simulink library "libbha_kinetic_cc"  (R2013b)
settings: Solver=FixedStepDiscrete  StartTime=0.0  StopTime=Inf  FixedStep=0.004  RelTol=1e-3
PostLoadFcn:
  | , if any(exist('dsrtsu_mdlpostloadfcn', 'file') == [2, 3, 6]), try dsrtsu_mdlpostloadfcn('Execute', bdroot); catch fprintf('Error in PostLoadFcn (dsrtsu_mdlpostloadfcn) for model "%s":\n %s\n', bdroot, lasterr); end, end,
libraries: libbha_parts_bellows x2
(part 2 of 4)

== matlab function libbha_kinetic_cc/lib_kinm_ext_S1 ==
  data: q input size=[3,1]; dq input size=[3,1]; H_1b_w input size=[4,4]; PAR_ell_ib input size=1; PAR_ell_ih input size=1; PAR_r_Bi input size=1; H_1h_w output size=[4,4]; dHdq_1h_w output size=[12,4]; dHPdq_1h_w output size=[12,4]; r_Bik_1h output size=[4,3]
% Kinetic Simulation
function [H_1h_w, dHdq_1h_w, dHPdq_1h_w, r_Bik_1h ] =  ksim_ext(q,dq, H_1b_w, PAR_ell_ib, PAR_ell_ih, PAR_r_Bi)

  
    
    % Änderungen zut alten Version:
    % - Rückrechnung mit Offsets der 4. Dimension der Homogenen Transformation (HOxx)
    % - richtige Saturierung des Ausgangsdrucks (optional)
    % - Tensordarstellung vermieden (Vektoren oder Matrizen sofern möglich), daher auch mehr getrennte Variablen
    % - Zusammenfassung bei Berechnungen unter Ausnutzung von 0-Einträgen (schwerer lesbar und weniger allgemein, dafür schneller zu rechnen)


%% Zustands- und Ableitungsberechnung der Homogenen Transformationen
    
    k                 = calc_k_i(q(1), q(2), q(3), PAR_r_Bi(1));
    
    dkdq_S1              = calc_dkdq_i(q(1), q(2), q(3), PAR_r_Bi(1));
	
	d2kdqdq_S1 	  = calc_d2kdqdq_i(q(1), q(2), q(3), PAR_r_Bi(1));
    
    % Relative Homogene Transformation und dessen Ableitung im lokalen Sektions-KoSy    
	[H_1h_1b, H_1b1, H_1h1] = calc_H_ih_ib(k(1), k(2), k(3), PAR_ell_ib(1), PAR_ell_ih(1));
    
    [dHdq_1h_1b, dHdk_1h_1b] = calc_dHdq_ih_ib(k(1), k(2), k(3), dkdq_S1, H_1b1, H_1h1);
	
    [d2Hdqdq_1h_1b, ~            ] = calc_d2Hdqdq_ih_ib(k(1), k(2), k(3), dkdq_S1, d2kdqdq_S1, dHdk_1h_1b, H_1b1, H_1h1);
    
    % Absolute Homogene Transformation und dessen Ableitung im Welt-KoSy
    H_1h_w = H_1b_w * H_1h_1b;
    
    dHdq_1h_w = zeros(4*3,4); % 4x4 Matrix abgeleitet nach 3 Zuständen q_i.
    dHdq_1h_w((1:12)   ,:) = MM(H_1b_w,dHdq_1h_1b);
	
	d2Hdqdq_1h_w = zeros(4*3,4*3);
	d2Hdqdq_1h_w((1:12)   ,(1:12)   ) = MM(H_1b_w, d2Hdqdq_1h_1b);
	
	dHPdq_1h_w = calc_dHPdq(d2Hdqdq_1h_w, dq); 
	
%% Kinetische Vorwärtsrechnung

    %r_S1_1h = [0;0;0;1];
    
    r_Bik_1h = [ PAR_r_Bi(1), -PAR_r_Bi(1)/2,         -PAR_r_Bi(1)/2;
				 0,            sqrt(3)/2*PAR_r_Bi(1),  -sqrt(3)/2*PAR_r_Bi(1)  
                 0, 0, 0; 1, 1, 1 ];

end

% ##################### Hilfsfunktionen #####################

%%  Konfigurationszustand k = [phi, kappa, ell]^T 

%  Konfigurationszustand einer Sektion 
function [k_i] = calc_k_i(q1,q2,q3, d)
    % Input:
    %   - qi = [ell_i1, ell_i2, ell_i3]^T       Aktorzustand
    %   - d                                     Radialer Abstand der Aktorsymmetrielinie  
    %
    % Output:
    %   - ki   [3 x 1]                          Konfigurationszustand 

    % Vermeidung Singularität
    qist_eps  = 1e-15;
    qist      = q1.^2 + q2.^2 + q3.^2 - q1.*q2 - q1.*q3 - q2.*q3;
    while (qist<qist_eps)
        q1      = q1 - 5e-8;
        qist  = q1.^2 + q2.^2 + q3.^2 - q1.*q2 - q1.*q3 - q2.*q3;
    end

    % Substitutionen
    q_sum   = q1 + q2 + q3;
    
    % Konfigurationszustand
    mphi    = atan2(sqrt(0.3e1) * (q3-q2) , (q2+q3 - 2*q1));
    mkappa  = 2.0 * sqrt(qist) / (d*q_sum);
    mell    = (q1 + q2 + q3)/3.0;
    
    k_i = [mphi;
           mkappa;
           mell];
end

% Partielle Ableitung 1. Ordnung nach q
function [dkdq_i] = calc_dkdq_i(q1,q2,q3, d)

    % Input:
	%   - qi = [ell_i1, ell_i2, ell_i3]^T       Aktorzustand
    %   - d                                     Radialer Abstand der Aktorsymmetrielinie
	%
	% Output:
	%   - dkdq_i   [3 x 3]                      Partielle Ableitung von Konfigurationszuständen ki nach Aktorzuständen qi 
 
    % Vermeidung Singularität
    qist_eps  = 1e-15;
    qist      = q1.^2 + q2.^2 + q3.^2 - q1.*q2 - q1.*q3 - q2.*q3;
    while (qist<qist_eps)
        q1      = q1-5e-8;
        qist  = q1.^2 + q2.^2 + q3.^2 - q1*q2 - q1*q3 - q2*q3;
    end

    % Substitutionen
    q_sum   = q1 + q2 + q3;

    % Ableitungen
    dkdq_i = zeros(3, 3);
    
    % dk1_dqb
    mdphi_dq1 =  sqrt(3.0) * ( q3 - q2) / qist / 2.0;
    mdphi_dq2 =  sqrt(3.0) * (-q3 + q1) / qist / 2.0;
    mdphi_dq3 = -sqrt(3.0) * (-q2 + q1) / qist / 2.0;
    
    dkdq_i(1, :) = [mdphi_dq1, mdphi_dq2, mdphi_dq3];
    
    % dk2_dqb
    mdkappa_dq1 =  3 * ( q2*q1 - q2^2  + q3*q1 - q3^2) / sqrt(qist) / d / q_sum^2;
    mdkappa_dq2 = -3 * (-q2*q1 - q2*q3 + q3^2  + q1^2) / sqrt(qist) / d / q_sum^2;
    mdkappa_dq3 = -3 * ( q2^2  - q2*q3 - q3*q1 + q1^2) / sqrt(qist) / d / q_sum^2;
    
    dkdq_i(2, :) = [mdkappa_dq1, mdkappa_dq2, mdkappa_dq3];
    
    % dk3_dqb
    mdell_dq1 = 1.0/3.0;
    mdell_dq2 = 1.0/3.0;
    mdell_dq3 = 1.0/3.0;
    
    dkdq_i(3, :) = [mdell_dq1, mdell_dq2, mdell_dq3];
end

function [d2kdqdq_i] = calc_d2kdqdq_i(q1,q2,q3, d)
% Input:
%   - qi = [ell_i1, ell_i2, ell_i3]^T       Aktorzustand
%
% Output:
%   - d2kdqdq_S1   [3*dim_qi x dim_qi]   Partielle Ableitung 2.Ord. von allen Konfigurationszuständen ki nach allen Aktorzuständen qi 
 
    % Vermeidung Singularität
    q_dist_eps  = 1e-15;
    q_dist      = q1 ^ 2 + q2 ^ 2 + q3 ^ 2 - q1 * q2 - q1 * q3 - q2 * q3;
    while (q_dist<q_dist_eps)
        q1      = q1-5e-8;
        q_dist  = q1 ^ 2 + q2 ^ 2 + q3 ^ 2 - q1 * q2 - q1 * q3 - q2 * q3;
    end

    % Substitutionen
    q_sum   = q1 + q2 + q3;

    % Ableitungen
    d2kdqdq_i = zeros(3*3, 3);
    
    % d2k1_dqbdqc
    mddphi_dq1dq1 = -sqrt(0.3e1) * (q3 - q2) / q_dist ^ 2 * (-q2 - q3 + 2 * q1) / 0.2e1;
    mddphi_dq1dq2 = -sqrt(0.3e1) * (-q2 ^ 2 + 2 * q2 * q3 - 2 * q3 * q1 + q1 ^ 2) / q_dist ^ 2 / 0.2e1;
    mddphi_dq1dq3 = sqrt(0.3e1) * (2 * q2 * q3 - 2 * q2 * q1 - q3 ^ 2 + q1 ^ 2) / q_dist ^ 2 / 0.2e1;
    
    mddphi_dq2dq1 = mddphi_dq1dq2;
    mddphi_dq2dq2 = sqrt(0.3e1) * (-q3 + q1) * (-2 * q2 + q3 + q1) / q_dist ^ 2 / 0.2e1;
    mddphi_dq2dq3 = -sqrt(0.3e1) * (q2 ^ 2 - 2 * q2 * q1 - q3 ^ 2 + 2 * q3 * q1) / q_dist ^ 2 / 0.2e1;
    
    mddphi_dq3dq1 = mddphi_dq1dq3;
    mddphi_dq3dq2 = mddphi_dq2dq3;
    mddphi_dq3dq3 = -sqrt(0.3e1) * (-q2 + q1) * (q2 - 2 * q3 + q1) / q_dist ^ 2 / 0.2e1;
    
    d2kdqdq_i([1, 4, 7], 1) = [mddphi_dq1dq1, mddphi_dq2dq1, mddphi_dq3dq1];
    d2kdqdq_i([1, 4, 7], 2) = [mddphi_dq1dq2, mddphi_dq2dq2, mddphi_dq3dq2];
    d2kdqdq_i([1, 4, 7], 3) = [mddphi_dq1dq3, mddphi_dq2dq3, mddphi_dq3dq3];
    
    % dk2_dqbdqc
    mddkappa_dq1dq1 = -0.3e1 / 0.2e1 * (-6 * q2 * q1 ^ 2 * q3 + 6 * q2 * q1 * q3 ^ 2 + 6 * q2 ^ 2 * q1 * q3 - 9 * q2 ^ 2 * q1 ^ 2 - 5 * q2 ^ 4 - 5 * q3 ^ 4 + 4 * q3 ^ 3 * q2 + 6 * q2 ^ 3 * q1 + 4 * q2 * q1 ^ 3 + 4 * q2 ^ 3 * q3 - 6 * q2 ^ 2 * q3 ^ 2 - 9 * q3 ^ 2 * q1 ^ 2 + 6 * q3 ^ 3 * q1 + 4 * q3 * q1 ^ 3) * (q_dist ^ (-0.3e1 / 0.2e1)) / d / (q_sum ^ 3);
    mddkappa_dq1dq2 = 0.3e1 / 0.2e1 * (2 * q2 ^ 4 + 3 * q3 ^ 4 + 3 * q2 * q1 ^ 2 * q3 + 3 * q2 ^ 2 * q1 * q3 - 3 * q2 * q1 * q3 ^ 2 + 6 * q2 ^ 2 * q1 ^ 2 - 7 * q2 ^ 3 * q1 - 7 * q2 * q1 ^ 3 - 3 * q2 ^ 3 * q3 + 9 * q2 ^ 2 * q3 ^ 2 - 3 * q3 * q1 ^ 3 + 9 * q3 ^ 2 * q1 ^ 2 - 7 * q3 ^ 3 * q2 - 7 * q3 ^ 3 * q1 + 2 * q1 ^ 4) * (q_dist ^ (-0.3e1 / 0.2e1)) / d / (q_sum ^ 3);
    mddkappa_dq1dq3 = 0.3e1 / 0.2e1 * (3 * q2 ^ 4 + 2 * q3 ^ 4 + 3 * q2 * q1 ^ 2 * q3 - 3 * q2 ^ 2 * q1 * q3 + 3 * q2 * q1 * q3 ^ 2 + 9 * q2 ^ 2 * q1 ^ 2 - 7 * q2 ^ 3 * q1 - 3 * q2 * q1 ^ 3 - 7 * q2 ^ 3 * q3 + 9 * q2 ^ 2 * q3 ^ 2 - 7 * q3 * q1 ^ 3 + 6 * q3 ^ 2 * q1 ^ 2 - 3 * q3 ^ 3 * q2 - 7 * q3 ^ 3 * q1 + 2 * q1 ^ 4) * (q_dist ^ (-0.3e1 / 0.2e1)) / d / (q_sum ^ 3);
    
    mddkappa_dq2dq1 = mddkappa_dq1dq2;
    mddkappa_dq2dq2 = 0.3e1 / 0.2e1 * (5 * q3 ^ 4 - 6 * q2 * q1 ^ 2 * q3 + 6 * q2 ^ 2 * q1 * q3 - 6 * q2 * q1 * q3 ^ 2 + 9 * q2 ^ 2 * q1 ^ 2 - 4 * q2 ^ 3 * q1 - 6 * q2 * q1 ^ 3 - 4 * q2 ^ 3 * q3 + 9 * q2 ^ 2 * q3 ^ 2 - 4 * q3 * q1 ^ 3 + 6 * q3 ^ 2 * q1 ^ 2 - 6 * q3 ^ 3 * q2 - 4 * q3 ^ 3 * q1 + 5 * q1 ^ 4) * (q_dist ^ (-0.3e1 / 0.2e1)) / d / (q_sum ^ 3);
    mddkappa_dq2dq3 = 0.3e1 / 0.2e1 * (2 * q2 ^ 4 + 2 * q3 ^ 4 - 3 * q2 * q1 ^ 2 * q3 + 3 * q2 ^ 2 * q1 * q3 + 3 * q2 * q1 * q3 ^ 2 + 9 * q2 ^ 2 * q1 ^ 2 - 3 * q2 ^ 3 * q1 - 7 * q2 ^ 3 * q3 + 6 * q2 ^ 2 * q3 ^ 2 - 7 * q2 * q3 ^ 3 - 3 * q3 ^ 3 * q1 + 9 * q3 ^ 2 * q1 ^ 2 - 7 * q1 ^ 3 * q3 - 7 * q1 ^ 3 * q2 + 3 * q1 ^ 4) * (q_dist ^ (-0.3e1 / 0.2e1)) / d / (q_sum ^ 3);

    mddkappa_dq3dq1 = mddkappa_dq1dq3;
    mddkappa_dq3dq2 = mddkappa_dq2dq3;
    mddkappa_dq3dq3 = 0.3e1 / 0.2e1 * (5 * q2 ^ 4 - 6 * q2 * q1 ^ 2 * q3 - 6 * q2 ^ 2 * q1 * q3 + 6 * q2 * q1 * q3 ^ 2 + 6 * q2 ^ 2 * q1 ^ 2 - 4 * q2 ^ 3 * q1 - 6 * q2 ^ 3 * q3 + 9 * q2 ^ 2 * q3 ^ 2 - 4 * q2 * q3 ^ 3 - 4 * q3 ^ 3 * q1 + 9 * q3 ^ 2 * q1 ^ 2 - 6 * q1 ^ 3 * q3 - 4 * q1 ^ 3 * q2 + 5 * q1 ^ 4) * (q_dist ^ (-0.3e1 / 0.2e1)) / d / (q_sum ^ 3);

    d2kdqdq_i([2, 5, 8], 1) = [mddkappa_dq1dq1, mddkappa_dq2dq1, mddkappa_dq3dq1];
    d2kdqdq_i([2, 5, 8], 2) = [mddkappa_dq1dq2, mddkappa_dq2dq2, mddkappa_dq3dq2];
    d2kdqdq_i([2, 5, 8], 3) = [mddkappa_dq1dq3, mddkappa_dq2dq3, mddkappa_dq3dq3];
    
    % dk3_dqbdqc
    % partielle Ableitungen 2. Ord von ell sind alle 0
end

%%  Homogene Transformationen 

%  Homogene Transformation 
%function [H_ih_ib] = calc_H_ih_ib(k1, k2, k3, PAR_ell_ib, PAR_ell_ih) 
function [H_ih_ib, H_im1_ib, H_ih_i] = calc_H_ih_ib(k1, k2, k3, PAR_ell_ib, PAR_ell_ih) 
    % Input:
    %   - ki = [phi, kappa, ell]^T              Konfigurationszustand
    %
    % Output:
    %   - H_i_im1   [4 x 4]                     Homogene Transformation
    
    % Vermeidung Singularität
    k2_eps = 1e-6;
    k2     = max([k2_eps, k2]);
    
    % Substitutionen
    sk1     = sin(k1);
    ck1     = cos(k1);
    sk2k3   = sin(k2 * k3);
    ck2k3   = cos(k2 * k3);
    
    % Trafo
    mHT_i_im1_11 = ck1 ^ 2 * (ck2k3 - 0.1e1) + 0.1e1;
    mHT_i_im1_12 = sk1 * ck1 * (ck2k3 - 0.1e1);
    mHT_i_im1_13 = ck1 * sk2k3;
    mHT_i_im1_14 = -ck1 * (ck2k3 - 0.1e1) / k2;
    
    mHT_i_im1_21 = sk1 * ck1 * (ck2k3 - 0.1e1);
    mHT_i_im1_22 = -ck1 ^ 2 * (ck2k3 - 0.1e1) + ck2k3;
    mHT_i_im1_23 = sk1 * sk2k3;
    mHT_i_im1_24 = -sk1 * (ck2k3 - 0.1e1) / k2;
    
    mHT_i_im1_31 = -ck1 * sk2k3;
    mHT_i_im1_32 = -sk1 * sk2k3;
    mHT_i_im1_33 = ck2k3;
    mHT_i_im1_34 = sk2k3 / k2;
    
    H_i_im1 = [mHT_i_im1_11, mHT_i_im1_12, mHT_i_im1_13, mHT_i_im1_14;
               mHT_i_im1_21, mHT_i_im1_22, mHT_i_im1_23, mHT_i_im1_24;
               mHT_i_im1_31, mHT_i_im1_32, mHT_i_im1_33, mHT_i_im1_34;
               0,            0,            0,            1            ];
           
    % Statische Begrenzungen
    H_im1_ib = eye(4);    
    H_ih_i   = eye(4);
    H_im1_ib(3,4) = PAR_ell_ib;
	H_ih_i(3,4)   = PAR_ell_ih;
    
    H_ih_ib = H_im1_ib * H_i_im1 * H_ih_i;
end

function [dHdk_i_i] = calc_dHdk_i_i(k1, k2, k3)
    % Input:
	%   - ki = [phi, kappa, ell]^T              Konfigurationszustand
	%
	% Output:
	%   - dH_i_in_im1_dka   [4*3x4]      Partielle Ableitung von H_i_in_im1 nach allen Konfigurationszuständen ki mit dim_ki=3
    
    % Vermeidung Singularität
    k2_eps = 1e-6;
    k2     = max([k2_eps, k2]);
    
    % Substitutionen
    sk1     = sin(k1);
    ck1     = cos(k1);
    sk2k3   = sin(k2 * k3);
    ck2k3   = cos(k2 * k3);
    
    dHdk_i_i = zeros(4*3, 4);
    
    % dHdk1_i_im1
    mdH_i_in_im1_dk1_11 = -2 * sk1 * ck1 * (ck2k3 - 1);
    mdH_i_in_im1_dk1_12 = 2 * ck2k3 * ck1 ^ 2 - ck2k3 - 2 * ck1 ^ 2 + 1;
    mdH_i_in_im1_dk1_13 = -sk1 * sk2k3;
    mdH_i_in_im1_dk1_14 = sk1 * (ck2k3 - 1) / k2;
    
    mdH_i_in_im1_dk1_21 = 2 * ck2k3 * ck1 ^ 2 - ck2k3 - 2 * ck1 ^ 2 + 1;
    mdH_i_in_im1_dk1_22 = 2 * sk1 * ck1 * (ck2k3 - 1);
    mdH_i_in_im1_dk1_23 = ck1 * sk2k3;
    mdH_i_in_im1_dk1_24 = -ck1 * (ck2k3 - 1) / k2;
    
    mdH_i_in_im1_dk1_31 = sk1 * sk2k3;
    mdH_i_in_im1_dk1_32 = -ck1 * sk2k3;
    mdH_i_in_im1_dk1_33 = 0;
    mdH_i_in_im1_dk1_34 = 0;
    
    dHdk_i_i(1:3,:) =         [mdH_i_in_im1_dk1_11, mdH_i_in_im1_dk1_12, mdH_i_in_im1_dk1_13, mdH_i_in_im1_dk1_14;
                               mdH_i_in_im1_dk1_21, mdH_i_in_im1_dk1_22, mdH_i_in_im1_dk1_23, mdH_i_in_im1_dk1_24;
                               mdH_i_in_im1_dk1_31, mdH_i_in_im1_dk1_32, mdH_i_in_im1_dk1_33, mdH_i_in_im1_dk1_34 ];
    
    % dHdk2_i_im1
    mdH_i_in_im1_dk2_11 = -ck1 ^ 2 * sk2k3 * k3;
    mdH_i_in_im1_dk2_12 = -sk1 * ck1 * sk2k3 * k3;
    mdH_i_in_im1_dk2_13 = ck1 * ck2k3 * k3;
    mdH_i_in_im1_dk2_14 = ck1 * (sk2k3 * k3 * k2 + ck2k3 - 1) / k2 ^ 2;
    
    mdH_i_in_im1_dk2_21 = -sk1 * ck1 * sk2k3 * k3;
    mdH_i_in_im1_dk2_22 = -sk2k3 * sk1 ^ 2 * k3;
    mdH_i_in_im1_dk2_23 = sk1 * ck2k3 * k3;
    mdH_i_in_im1_dk2_24 = sk1 * (sk2k3 * k3 * k2 + ck2k3 - 1) / k2 ^ 2;
    
    mdH_i_in_im1_dk2_31 = -ck1 * ck2k3 * k3;
    mdH_i_in_im1_dk2_32 = -sk1 * ck2k3 * k3;
    mdH_i_in_im1_dk2_33 = -sk2k3 * k3;
    mdH_i_in_im1_dk2_34 = (ck2k3 * k3 * k2 - sk2k3) / k2 ^ 2;
    
    dHdk_i_i(5:7,:) =         [mdH_i_in_im1_dk2_11, mdH_i_in_im1_dk2_12, mdH_i_in_im1_dk2_13, mdH_i_in_im1_dk2_14;
                               mdH_i_in_im1_dk2_21, mdH_i_in_im1_dk2_22, mdH_i_in_im1_dk2_23, mdH_i_in_im1_dk2_24;
                               mdH_i_in_im1_dk2_31, mdH_i_in_im1_dk2_32, mdH_i_in_im1_dk2_33, mdH_i_in_im1_dk2_34 ];
    
    % dHdk3_i_im1
    mdH_i_in_im1_dk3_11 = -ck1 ^ 2 * sk2k3 * k2;
    mdH_i_in_im1_dk3_12 = -sk1 * ck1 * sk2k3 * k2;
    mdH_i_in_im1_dk3_13 = ck1 * ck2k3 * k2;
    mdH_i_in_im1_dk3_14 = ck1 * sk2k3;
    
    mdH_i_in_im1_dk3_21 = -sk1 * ck1 * sk2k3 * k2;
    mdH_i_in_im1_dk3_22 = -sk2k3 * sk1 ^ 2 * k2;
    mdH_i_in_im1_dk3_23 = sk1 * ck2k3 * k2;
    mdH_i_in_im1_dk3_24 = sk1 * sk2k3;
    
    mdH_i_in_im1_dk3_31 = -ck1 * ck2k3 * k2;
    mdH_i_in_im1_dk3_32 = -sk1 * ck2k3 * k2;
    mdH_i_in_im1_dk3_33 = -sk2k3 * k2;
    mdH_i_in_im1_dk3_34 = ck2k3;
    
    dHdk_i_i(9:11,:) =        [mdH_i_in_im1_dk3_11, mdH_i_in_im1_dk3_12, mdH_i_in_im1_dk3_13, mdH_i_in_im1_dk3_14;
                               mdH_i_in_im1_dk3_21, mdH_i_in_im1_dk3_22, mdH_i_in_im1_dk3_23, mdH_i_in_im1_dk3_24;
                               mdH_i_in_im1_dk3_31, mdH_i_in_im1_dk3_32, mdH_i_in_im1_dk3_33, mdH_i_in_im1_dk3_34 ];
end

%function [dHdq_ih_ib, dHdk_ih_ib] = calc_dHdq_ih_ib(k1, k2, k3, dkdq_i, PAR_ell_ib, PAR_ell_ih)
function [dHdq_ih_ib, dHdk_ih_ib] = calc_dHdq_ih_ib(k1, k2, k3, dkdq_i, H_ibi, H_ihi)

    % Input:
	%   - ki = [phi, kappa, ell]^T              Konfigurationszustand
	%   - dkdq_i            [3=dim_kix3=dim_qi] Partielle Ableitung von allen Konfigurationszuständen ki nach allen Aktorzuständen qi 
	%
	% Output:
	%   - dH_i_in_im1_dqa   [4*3x4]      Partielle Ableitung von H_ih_ib nach allen Aktorzuständen qi mit dim_di = 3

    dHdq_ih_ib = zeros(4*3,4);

    % Statische Begrenzungen
    %H_im1_ib = eye(4);    
    %H_ih_i   = eye(4);
    %H_im1_ib(3,4) = PAR_ell_ib;
	%H_ih_i(3,4)   = PAR_ell_ih;
    
    % Kettenregel
    dHdk_ih_ib = calc_dHdk_i_i(k1, k2, k3);
    for j=1:3
		jm = j-1;
		%dHdq_ih_ib((1:4)+jm*4,:) = H_im1_ib * (dHdk_ih_ib(1:4,:).*dkdq_i(1,j) + dHdk_ih_ib(5:8,:).*dkdq_i(2,j) + dHdk_ih_ib(9:12,:).*dkdq_i(3,j)) * H_ih_i; % H_base * ( dHdq_i_i ) * H_head // mit dHdq_i_i = dH/dk1 * dk1/dqj + dH/dk2 * dk2/dqj + dH/dk3 * dk3/dqj
		dHdq_ih_ib((1:4)+jm*4,:) = H_ibi * (dHdk_ih_ib(1:4,:).*dkdq_i(1,j) + dHdk_ih_ib(5:8,:).*dkdq_i(2,j) + dHdk_ih_ib(9:12,:).*dkdq_i(3,j)) * H_ihi; % H_base * ( dHdq_i_i ) * H_head // mit dHdq_i_i = dH/dk1 * dk1/dqj + dH/dk2 * dk2/dqj + dH/dk3 * dk3/dqj
    end
end

function d2Hdkdk_ih_ib = calc_d2Hdkdk_ih_ib(k1, k2, k3)
% Input:
%   - ki = [phi, kappa, ell]^T              Konfigurationszustand
%
% Output
%   - d2Hdkdk_ih_ib   [4*dim_ki x 4*dim_ki]       Partielle Ableitung 2.Ord von H_i_in_im1 nach allen Konfigurationszuständen ki 
    
    % Vermeidung Singularität
    k2_eps = 1e-6;
    k2     = max([k2_eps, k2]);
    
    % Substitutionen
    sk1     = sin(k1);
    ck1     = cos(k1);
    sk2k3   = sin(k2 * k3);
    ck2k3   = cos(k2 * k3);
    
    dim_ki = 3;
    d2Hdkdk_ih_ib = zeros(4*dim_ki, 4*dim_ki);
    
% d2H_i_in_im1_dk1dk1
    mddH_i_in_im1_dk1dk1_11 = -0.4e1 * ck2k3 * ck1 ^ 2 + 0.2e1 * ck2k3 + 0.4e1 * ck1 ^ 2 - 0.2e1;
    mddH_i_in_im1_dk1dk1_12 = -0.4e1 * sk1 * ck1 * (ck2k3 - 0.1e1);
    mddH_i_in_im1_dk1dk1_13 = -ck1 * sk2k3;
    mddH_i_in_im1_dk1dk1_14 = ck1 * (ck2k3 - 0.1e1) / k2;
    
    mddH_i_in_im1_dk1dk1_21 = -0.4e1 * sk1 * ck1 * (ck2k3 - 0.1e1);
    mddH_i_in_im1_dk1dk1_22 = 0.4e1 * ck2k3 * ck1 ^ 2 - 0.2e1 * ck2k3 - 0.4e1 * ck1 ^ 2 + 0.2e1;
    mddH_i_in_im1_dk1dk1_23 = -sk1 * sk2k3;
    mddH_i_in_im1_dk1dk1_24 = sk1 * (ck2k3 - 0.1e1) / k2;
    
    mddH_i_in_im1_dk1dk1_31 = ck1 * sk2k3;
    mddH_i_in_im1_dk1dk1_32 = sk1 * sk2k3;
    mddH_i_in_im1_dk1dk1_33 = 0;
    mddH_i_in_im1_dk1dk1_34 = 0;
    
    d2Hdkdk_ih_ib(1:3, 1:4)       = [mddH_i_in_im1_dk1dk1_11, mddH_i_in_im1_dk1dk1_12, mddH_i_in_im1_dk1dk1_13, mddH_i_in_im1_dk1dk1_14;
                                           mddH_i_in_im1_dk1dk1_21, mddH_i_in_im1_dk1dk1_22, mddH_i_in_im1_dk1dk1_23, mddH_i_in_im1_dk1dk1_24;
                                           mddH_i_in_im1_dk1dk1_31, mddH_i_in_im1_dk1dk1_32, mddH_i_in_im1_dk1dk1_33, mddH_i_in_im1_dk1dk1_34 ]; 
    
    
    % d2H_i_in_im1_dk2dk2
    mddH_i_in_im1_dk2dk2_11 = -ck1 ^ 2 * ck2k3 * k3 ^ 2;
    mddH_i_in_im1_dk2dk2_12 = -sk1 * ck1 * ck2k3 * k3 ^ 2;
    mddH_i_in_im1_dk2dk2_13 = -ck1 * sk2k3 * k3 ^ 2;
    mddH_i_in_im1_dk2dk2_14 = -ck1 * (-ck2k3 * k3 ^ 2 * k2 ^ 2 + 0.2e1 * sk2k3 * k3 * k2 + 0.2e1 * ck2k3 - 0.2e1) / k2 ^ 3;
    
    mddH_i_in_im1_dk2dk2_21 = -sk1 * ck1 * ck2k3 * k3 ^ 2;
    mddH_i_in_im1_dk2dk2_22 = -ck2k3 * k3 ^ 2 * sk1 ^ 2;
    mddH_i_in_im1_dk2dk2_23 = -sk1 * sk2k3 * k3 ^ 2;
    mddH_i_in_im1_dk2dk2_24 = -sk1 * (-ck2k3 * k3 ^ 2 * k2 ^ 2 + 0.2e1 * sk2k3 * k3 * k2 + 0.2e1 * ck2k3 - 0.2e1) / k2 ^ 3;
    
    mddH_i_in_im1_dk2dk2_31 = ck1 * sk2k3 * k3 ^ 2;
    mddH_i_in_im1_dk2dk2_32 = sk1 * sk2k3 * k3 ^ 2;
    mddH_i_in_im1_dk2dk2_33 = -ck2k3 * k3 ^ 2;
    mddH_i_in_im1_dk2dk2_34 = -(sk2k3 * k3 ^ 2 * k2 ^ 2 + 0.2e1 * ck2k3 * k3 * k2 - 0.2e1 * sk2k3) / k2 ^ 3;
    
    d2Hdkdk_ih_ib(5:7, 5:8)       = [mddH_i_in_im1_dk2dk2_11, mddH_i_in_im1_dk2dk2_12, mddH_i_in_im1_dk2dk2_13, mddH_i_in_im1_dk2dk2_14;
                                           mddH_i_in_im1_dk2dk2_21, mddH_i_in_im1_dk2dk2_22, mddH_i_in_im1_dk2dk2_23, mddH_i_in_im1_dk2dk2_24;
                                           mddH_i_in_im1_dk2dk2_31, mddH_i_in_im1_dk2dk2_32, mddH_i_in_im1_dk2dk2_33, mddH_i_in_im1_dk2dk2_34 ]; 
                                       
    % d2H_i_in_im1_dk3dk3
    mddH_i_in_im1_dk3dk3_11 = -ck1 ^ 2 * ck2k3 * k2 ^ 2;
    mddH_i_in_im1_dk3dk3_12 = -sk1 * ck1 * ck2k3 * k2 ^ 2;
    mddH_i_in_im1_dk3dk3_13 = -ck1 * sk2k3 * k2 ^ 2;
    mddH_i_in_im1_dk3dk3_14 = ck1 * ck2k3 * k2;
    
    mddH_i_in_im1_dk3dk3_21 = -sk1 * ck1 * ck2k3 * k2 ^ 2;
    mddH_i_in_im1_dk3dk3_22 = -ck2k3 * k2 ^ 2 * sk1 ^ 2;
    mddH_i_in_im1_dk3dk3_23 = -sk1 * sk2k3 * k2 ^ 2;
    mddH_i_in_im1_dk3dk3_24 = sk1 * ck2k3 * k2;
    
    mddH_i_in_im1_dk3dk3_31 = ck1 * sk2k3 * k2 ^ 2;
    mddH_i_in_im1_dk3dk3_32 = sk1 * sk2k3 * k2 ^ 2;
    mddH_i_in_im1_dk3dk3_33 = -ck2k3 * k2 ^ 2;
    mddH_i_in_im1_dk3dk3_34 = -sk2k3 * k2;
    
    d2Hdkdk_ih_ib(9:11, 9:12)     = [mddH_i_in_im1_dk3dk3_11, mddH_i_in_im1_dk3dk3_12, mddH_i_in_im1_dk3dk3_13, mddH_i_in_im1_dk3dk3_14;
                                           mddH_i_in_im1_dk3dk3_21, mddH_i_in_im1_dk3dk3_22, mddH_i_in_im1_dk3dk3_23, mddH_i_in_im1_dk3dk3_24;
                                           mddH_i_in_im1_dk3dk3_31, mddH_i_in_im1_dk3dk3_32, mddH_i_in_im1_dk3dk3_33, mddH_i_in_im1_dk3dk3_34 ]; 
                                       
    % d2H_i_in_im1_dk1dk2 = d2H_i_in_im1_dk2dk1
    mddH_i_in_im1_dk1dk2_11 = 0.2e1 * sk1 * ck1 * sk2k3 * k3;
    mddH_i_in_im1_dk1dk2_12 = -sk2k3 * k3 * (0.2e1 * ck1 ^ 2 - 0.1e1);
    mddH_i_in_im1_dk1dk2_13 = -sk1 * ck2k3 * k3;
    mddH_i_in_im1_dk1dk2_14 = -sk1 * (sk2k3 * k3 * k2 + ck2k3 - 0.1e1) / k2 ^ 2;
    
    mddH_i_in_im1_dk1dk2_21 = -sk2k3 * k3 * (0.2e1 * ck1 ^ 2 - 0.1e1);
    mddH_i_in_im1_dk1dk2_22 = -0.2e1 * sk1 * ck1 * sk2k3 * k3;
    mddH_i_in_im1_dk1dk2_23 = ck1 * ck2k3 * k3;
    mddH_i_in_im1_dk1dk2_24 = ck1 * (sk2k3 * k3 * k2 + ck2k3 - 0.1e1) / k2 ^ 2;
    
    mddH_i_in_im1_dk1dk2_31 = sk1 * ck2k3 * k3;
    mddH_i_in_im1_dk1dk2_32 = -ck1 * ck2k3 * k3;
    mddH_i_in_im1_dk1dk2_33 = 0;
    mddH_i_in_im1_dk1dk2_34 = 0;
    
    d2Hdkdk_ih_ib(1:3, 5:8)       = [mddH_i_in_im1_dk1dk2_11, mddH_i_in_im1_dk1dk2_12, mddH_i_in_im1_dk1dk2_13, mddH_i_in_im1_dk1dk2_14;
                                           mddH_i_in_im1_dk1dk2_21, mddH_i_in_im1_dk1dk2_22, mddH_i_in_im1_dk1dk2_23, mddH_i_in_im1_dk1dk2_24;
                                           mddH_i_in_im1_dk1dk2_31, mddH_i_in_im1_dk1dk2_32, mddH_i_in_im1_dk1dk2_33, mddH_i_in_im1_dk1dk2_34 ]; 
    d2Hdkdk_ih_ib(5:7, 1:4) = d2Hdkdk_ih_ib(1:3, 5:8);
    
    % d2H_i_in_im1_dk1dk3 = d2H_i_in_im1_dk3dk1
    mddH_i_in_im1_dk1dk3_11 = 0.2e1 * sk1 * ck1 * sk2k3 * k2;
    mddH_i_in_im1_dk1dk3_12 = -sk2k3 * k2 * (0.2e1 * ck1 ^ 2 - 0.1e1);
    mddH_i_in_im1_dk1dk3_13 = -sk1 * ck2k3 * k2;
    mddH_i_in_im1_dk1dk3_14 = -sk1 * sk2k3;
    
    mddH_i_in_im1_dk1dk3_21 = -sk2k3 * k2 * (0.2e1 * ck1 ^ 2 - 0.1e1);
    mddH_i_in_im1_dk1dk3_22 = -0.2e1 * sk1 * ck1 * sk2k3 * k2;
    mddH_i_in_im1_dk1dk3_23 = ck1 * ck2k3 * k2;
    mddH_i_in_im1_dk1dk3_24 = ck1 * sk2k3;
    
    mddH_i_in_im1_dk1dk3_31 = sk1 * ck2k3 * k2;
    mddH_i_in_im1_dk1dk3_32 = -ck1 * ck2k3 * k2;
    mddH_i_in_im1_dk1dk3_33 = 0;
    mddH_i_in_im1_dk1dk3_34 = 0;
    
    d2Hdkdk_ih_ib(1:3, 9:12)      = [mddH_i_in_im1_dk1dk3_11, mddH_i_in_im1_dk1dk3_12, mddH_i_in_im1_dk1dk3_13, mddH_i_in_im1_dk1dk3_14;
                                           mddH_i_in_im1_dk1dk3_21, mddH_i_in_im1_dk1dk3_22, mddH_i_in_im1_dk1dk3_23, mddH_i_in_im1_dk1dk3_24;
                                           mddH_i_in_im1_dk1dk3_31, mddH_i_in_im1_dk1dk3_32, mddH_i_in_im1_dk1dk3_33, mddH_i_in_im1_dk1dk3_34 ]; 
    d2Hdkdk_ih_ib(9:11, 1:4) = d2Hdkdk_ih_ib(1:3, 9:12);
    
    % d2H_i_in_im1_dk2dk3 = d2H_i_in_im1_dk3dk2
    mddH_i_in_im1_dk2dk3_11 = -ck1 ^ 2 * (ck2k3 * k3 * k2 + sk2k3);
    mddH_i_in_im1_dk2dk3_12 = -sk1 * ck1 * (ck2k3 * k3 * k2 + sk2k3);
    mddH_i_in_im1_dk2dk3_13 = ck1 * (-sk2k3 * k3 * k2 + ck2k3);
    mddH_i_in_im1_dk2dk3_14 = ck1 * ck2k3 * k3;
    
    mddH_i_in_im1_dk2dk3_21 = -sk1 * ck1 * (ck2k3 * k3 * k2 + sk2k3);
    mddH_i_in_im1_dk2dk3_22 = -sk1 ^ 2 * (ck2k3 * k3 * k2 + sk2k3);
    mddH_i_in_im1_dk2dk3_23 = sk1 * (-sk2k3 * k3 * k2 + ck2k3);
    mddH_i_in_im1_dk2dk3_24 = sk1 * ck2k3 * k3;
    
    mddH_i_in_im1_dk2dk3_31 = -ck1 * (-sk2k3 * k3 * k2 + ck2k3);
    mddH_i_in_im1_dk2dk3_32 = -sk1 * (-sk2k3 * k3 * k2 + ck2k3);
    mddH_i_in_im1_dk2dk3_33 = -ck2k3 * k3 * k2 - sk2k3;
    mddH_i_in_im1_dk2dk3_34 = -sk2k3 * k3;
    
    d2Hdkdk_ih_ib(5:7, 9:12)      = [mddH_i_in_im1_dk2dk3_11, mddH_i_in_im1_dk2dk3_12, mddH_i_in_im1_dk2dk3_13, mddH_i_in_im1_dk2dk3_14;
                                           mddH_i_in_im1_dk2dk3_21, mddH_i_in_im1_dk2dk3_22, mddH_i_in_im1_dk2dk3_23, mddH_i_in_im1_dk2dk3_24;
                                           mddH_i_in_im1_dk2dk3_31, mddH_i_in_im1_dk2dk3_32, mddH_i_in_im1_dk2dk3_33, mddH_i_in_im1_dk2dk3_34 ]; 
    d2Hdkdk_ih_ib(9:11, 5:8) = d2Hdkdk_ih_ib(5:7, 9:12);
end

%function [d2Hdqdq_ih_ib, d2Hdkdk_ih_ib] = calc_d2Hdqdq_ih_ib(k1, k2, k3, dkdq_i, d2kdqdq_i, dHdk_ih_ib)
function [d2Hdqdq_ih_ib, d2Hdkdk_ih_ib] = calc_d2Hdqdq_ih_ib(k1, k2, k3, dkdq_i, d2kdqdq_i, dHdk_ih_ib, H_ibi, H_ihi)
	% Input:
%   - dkdqb_i               [3 x 3]           Partielle Ableitung von allen Konfigurationszuständen ki nach allen Aktorzuständen qi 
%   - d2kdqdq_i             [3*3 x 3]         Partielle Ableitung 2.Ord von allen Konfigurationszuständen ki nach allen Aktorzuständen qi 
%   - dHdk_ih_ib            [4*3 x 4]         Partielle Ableitung von H_ih_ib nach allen Konfigurationszuständen ki 
%
% Output:
%   - d2Hdqdq_ih_ib         [4*3 x 4*3]       Partielle Ableitung 2.Ord von H_ih_ib nach allen Aktorzuständen qi 
%   - d2Hdkdk_ih_ib		    [4*3 x 4*3]       Partielle Ableitung 2.Ord von H_ih_ib nach allen Konfigurationszuständen ki 
    
	d2Hdkdk_ih_ib = calc_d2Hdkdk_ih_ib(k1, k2, k3);
    
    d2Hdqdq_ih_ib = zeros(4*3, 4*3);
    for a = 1:3 % dim_qi
        for b = 1:3 % dim_qi
            for xi = 1:3 % dim_ki
                for chi = 1:3 % dim_ki
                    d2Hdqdq_ih_ib((1:4)+4*(a-1), (1:4)+4*(b-1)) = d2Hdqdq_ih_ib((1:4)+4*(a-1), (1:4)+4*(b-1)) + d2Hdkdk_ih_ib((1:4)+4*(xi-1), (1:4)+4*(chi-1)) * dkdq_i(chi, b) * dkdq_i(xi, a);					
                end
                d2Hdqdq_ih_ib((1:4)+4*(a-1), (1:4)+4*(b-1))     = d2Hdqdq_ih_ib((1:4)+4*(a-1), (1:4)+4*(b-1)) + dHdk_ih_ib((1:4)+4*(xi-1), :) * d2kdqdq_i(xi+3*(a-1), b);
            end
        end
    end
	d2Hdqdq_ih_ib = MM(MM(H_ibi,d2Hdqdq_ih_ib),H_ihi);
end

function [dHdt] = calc_HP(dHdq, dqdt)
% Input:
%   - dHdq    [4*dim_qi x 4]      Partielle Ableitung von H nach allen Aktorzuständen qi 
%   - dqdt    [dim_qi x 1]        Zeitableitung von allen Aktorzuständen qi 
%
% Output:
%   - dHdt    [4 x 4]             Zeitableitung von H 
    
   	dim_qi = size(dqdt, 1); %dim_qi = size(dHdq, 1)/4;
	
    dHdt = zeros(4, 4);
    for xi = 1:dim_qi
        dHdt =  dHdt + dHdq((1:4)+4*(xi-1),:)*dqdt(xi);        
    end
end

function [dHPdq] = calc_dHPdq(d2Hdqdq, dqdt) % Partielle Ableitung der Zeitableitung von H
% Input:
%   - d2Hdqdq    [4*dim_qi x 4*dim_qi]   Partielle Ableitung 2.Ord von H nach allen Aktorzuständen qi 
%   - dqdt       [dim_qi x 1]            Zeitableitung von allen Aktorzuständen qi 
%
% Output:
%   - dHPdq       [4*dim_qi x 4]          Partielle Ableitung nach allen Aktorzuständen qi der Zeitableitung von H 
    
    dim_qi = size(dqdt, 1);
    
    dHPdq = zeros(4*dim_qi, 4);
    for a = 1:dim_qi
        for xi = 1:dim_qi
            dHPdq((1:4)+4*(a-1),:) = dHPdq((1:4)+4*(a-1),:)...
                                      +d2Hdqdq((1:4)+4*(a-1),(1:4)+4*(xi-1))*dqdt(xi);
        end
    end
end


%% Matrix Helpers

function [H_2_0] = MMM(H_1_0, H_2_1) % Multiple Matrix Multiplication (Tensormultiplikation) für 4x4 * 4x4xn oder 4x4xn * 4x4

    H1_d3 = size(H_1_0,3);
    H2_d3 = size(H_2_1,3);
    H_2_0 = zeros(4,4,max(H1_d3,H2_d3));
    
    if H1_d3 == H2_d3
        for i=1:H2_d3
            H_2_0(:,:,i) = H_1_0(:,:,i) * H_2_1(:,:,i);
        end
    elseif H1_d3 == 1 && H2_d3 > 1
        for i=1:H2_d3
            H_2_0(:,:,i) = H_1_0 * H_2_1(:,:,i);
        end
    elseif H1_d3 > 1 && H2_d3 == 1
        for i=1:H1_d3
            H_2_0(:,:,i) = H_1_0(:,:,i) * H_2_1;
        end
    else
        error('case not handled here');
    end
end

function [H_2_0] = MM(H_1_0, H_2_1) % Matrix Multiplikation für 4x4 * 4nzx4ns
	% Input:
	%   - Eine Matrix [4x4]
	%   - Eine Matrix [4*nz x 4*ns]
	%
	% Output:
	%   - H_2_in_0 [4*n x 4*ns] = H_1_in_0*H_2_in_1

	[nz1, ns1] = size(H_1_0);
	[nz2, ns2] = size(H_2_1);

	nz_max = max(nz1./4, nz2./4);
	ns_max = max(ns1./4, ns2./4);

	H_2_0 = zeros(4*nz_max, 4*ns_max);

	if (nz1+ns1) < (nz2+ns2)
		for zz = 1:nz_max
			for ss = 1:ns_max
				H_2_0((1:4)+4*(zz-1), (1:4)+4*(ss-1)) = H_1_0 * H_2_1((1:4)+4*(zz-1), (1:4)+4*(ss-1));
			end
		end
	else
		for zz = 1:nz_max
			for ss = 1:ns_max
				H_2_0((1:4)+4*(zz-1), (1:4)+4*(ss-1)) = H_1_0((1:4)+4*(zz-1), (1:4)+4*(ss-1)) * H_2_1;
			end
		end
	end
end

function At = transpose4x4(A)
	% Input:
	%   - A     [4*z x 4*s]
	%
	% Output:
	%   - At    [4*s x 4*z]
	%
	% Bsp:
	% A = [a11, a12, a13, a14, b11, b12, b13, b14
	%      a21, a22, a23, a24, b21, b22, b23, b24
	%      a31, a32, a33, a34, b31, b32, b33, b34
	%      a41, a42, a43, a44, b41, b42, b43, b44];
	%
	% At =[a11, a12, a13, a14 
	%      a21, a22, a23, a24 
	%      a31, a32, a33, a34 
	%      a41, a42, a43, a44
	%      b11, b12, b13, b14
	%      b21, b22, b23, b24
	%      b31, b32, b33, b34
	%      b41, b42, b43, b44];

	At = zeros(size(A))';
	dim_z = size(A, 1)/4;
	dim_s = size(A, 2)/4;

	for iz = 1:dim_z
		for is = 1:dim_s
			At((1:4)+4*(is-1), (1:4)+4*(iz-1)) = A((1:4)+4*(iz-1), (1:4)+4*(is-1));
		end
	end
end

== matlab function libbha_kinetic_cc/lib_revkin_inhom ==
  data: H_1h_w input size=[4,4]; H_2h_w input size=[4,4]; H_3h_w input size=[4,4]; dHdq_1h_w input size=[36,4]; dHdq_2h_w input size=[36,4]; dHdq_3h_w input size=[36,4]; r_Bik_1h input size=[4,3]; rHinv output size=[9,9]; r_Bik_2h input size=[4,3]; r_Bik_3h input size=[4,3]; rH output size=[9,9]
function [rHinv, rH]   = ksim_rev_tinv(H_1h_w, H_2h_w, H_3h_w, dHdq_1h_w, dHdq_2h_w, dHdq_3h_w, r_Bik_1h, r_Bik_2h, r_Bik_3h)
% kinvsim_fav_4c

    % Herleitung: Review 2014
    % pd = 1/AP * Hinv * tau_d + pAmb
    % tau_d: Anteile der Mechanik-DGL (anteilig)
    

    %% Htilde
    
    HF11 = [H_1h_w(:,3)'*dHdq_1h_w( 1: 4,:)*r_Bik_1h(:,1), H_1h_w(:,3)'*dHdq_1h_w( 1: 4,:)*r_Bik_1h(:,2), H_1h_w(:,3)'*dHdq_1h_w( 1: 4,:)*r_Bik_1h(:,3) ;
            H_1h_w(:,3)'*dHdq_1h_w( 5: 8,:)*r_Bik_1h(:,1), H_1h_w(:,3)'*dHdq_1h_w( 5: 8,:)*r_Bik_1h(:,2), H_1h_w(:,3)'*dHdq_1h_w( 5: 8,:)*r_Bik_1h(:,3) ;
            H_1h_w(:,3)'*dHdq_1h_w( 9:12,:)*r_Bik_1h(:,1), H_1h_w(:,3)'*dHdq_1h_w( 9:12,:)*r_Bik_1h(:,2), H_1h_w(:,3)'*dHdq_1h_w( 9:12,:)*r_Bik_1h(:,3)   ];
        
	HF21 = [H_2h_w(:,3)'*dHdq_2h_w( 1: 4,:)*r_Bik_2h(:,1), H_2h_w(:,3)'*dHdq_2h_w( 1: 4,:)*r_Bik_2h(:,2), H_2h_w(:,3)'*dHdq_2h_w( 1: 4,:)*r_Bik_2h(:,3) ;
            H_2h_w(:,3)'*dHdq_2h_w( 5: 8,:)*r_Bik_2h(:,1), H_2h_w(:,3)'*dHdq_2h_w( 5: 8,:)*r_Bik_2h(:,2), H_2h_w(:,3)'*dHdq_2h_w( 5: 8,:)*r_Bik_2h(:,3) ;
            H_2h_w(:,3)'*dHdq_2h_w( 9:12,:)*r_Bik_2h(:,1), H_2h_w(:,3)'*dHdq_2h_w( 9:12,:)*r_Bik_2h(:,2), H_2h_w(:,3)'*dHdq_2h_w( 9:12,:)*r_Bik_2h(:,3)   ];      
    HF22 = [H_2h_w(:,3)'*dHdq_2h_w(13:16,:)*r_Bik_2h(:,1), H_2h_w(:,3)'*dHdq_2h_w(13:16,:)*r_Bik_2h(:,2), H_2h_w(:,3)'*dHdq_2h_w(13:16,:)*r_Bik_2h(:,3) ;
            H_2h_w(:,3)'*dHdq_2h_w(17:20,:)*r_Bik_2h(:,1), H_2h_w(:,3)'*dHdq_2h_w(17:20,:)*r_Bik_2h(:,2), H_2h_w(:,3)'*dHdq_2h_w(17:20,:)*r_Bik_2h(:,3) ;
            H_2h_w(:,3)'*dHdq_2h_w(21:24,:)*r_Bik_2h(:,1), H_2h_w(:,3)'*dHdq_2h_w(21:24,:)*r_Bik_2h(:,2), H_2h_w(:,3)'*dHdq_2h_w(21:24,:)*r_Bik_2h(:,3)   ];

    HF31 = [H_3h_w(:,3)'*dHdq_3h_w( 1: 4,:)*r_Bik_3h(:,1), H_3h_w(:,3)'*dHdq_3h_w( 1: 4,:)*r_Bik_3h(:,2), H_3h_w(:,3)'*dHdq_3h_w( 1: 4,:)*r_Bik_3h(:,3) ;
            H_3h_w(:,3)'*dHdq_3h_w( 5: 8,:)*r_Bik_3h(:,1), H_3h_w(:,3)'*dHdq_3h_w( 5: 8,:)*r_Bik_3h(:,2), H_3h_w(:,3)'*dHdq_3h_w( 5: 8,:)*r_Bik_3h(:,3) ;
            H_3h_w(:,3)'*dHdq_3h_w( 9:12,:)*r_Bik_3h(:,1), H_3h_w(:,3)'*dHdq_3h_w( 9:12,:)*r_Bik_3h(:,2), H_3h_w(:,3)'*dHdq_3h_w( 9:12,:)*r_Bik_3h(:,3)   ];
	HF32 = [H_3h_w(:,3)'*dHdq_3h_w(13:16,:)*r_Bik_3h(:,1), H_3h_w(:,3)'*dHdq_3h_w(13:16,:)*r_Bik_3h(:,2), H_3h_w(:,3)'*dHdq_3h_w(13:16,:)*r_Bik_3h(:,3) ;
            H_3h_w(:,3)'*dHdq_3h_w(17:20,:)*r_Bik_3h(:,1), H_3h_w(:,3)'*dHdq_3h_w(17:20,:)*r_Bik_3h(:,2), H_3h_w(:,3)'*dHdq_3h_w(17:20,:)*r_Bik_3h(:,3) ;
            H_3h_w(:,3)'*dHdq_3h_w(21:24,:)*r_Bik_3h(:,1), H_3h_w(:,3)'*dHdq_3h_w(21:24,:)*r_Bik_3h(:,2), H_3h_w(:,3)'*dHdq_3h_w(21:24,:)*r_Bik_3h(:,3)   ];  
	HF33 = [H_3h_w(:,3)'*dHdq_3h_w(25:28,:)*r_Bik_3h(:,1), H_3h_w(:,3)'*dHdq_3h_w(25:28,:)*r_Bik_3h(:,2), H_3h_w(:,3)'*dHdq_3h_w(25:28,:)*r_Bik_3h(:,3) ;
            H_3h_w(:,3)'*dHdq_3h_w(29:32,:)*r_Bik_3h(:,1), H_3h_w(:,3)'*dHdq_3h_w(29:32,:)*r_Bik_3h(:,2), H_3h_w(:,3)'*dHdq_3h_w(29:32,:)*r_Bik_3h(:,3) ; 
            H_3h_w(:,3)'*dHdq_3h_w(33:36,:)*r_Bik_3h(:,1), H_3h_w(:,3)'*dHdq_3h_w(33:36,:)*r_Bik_3h(:,2), H_3h_w(:,3)'*dHdq_3h_w(33:36,:)*r_Bik_3h(:,3)   ];
    
    rHtilde = [HF11, HF21, HF31; zeros(3), HF22, HF32; zeros(3,6), HF33];
    
    %% Hhat
    
    rHhat = eye(9)+[zeros(6,3),eye(6);zeros(3,9)]+[zeros(3,6),eye(3);zeros(6,9)];
    rHhatinv = eye(9)-[zeros(6,3),eye(6);zeros(3,9)];

    %% Zusammenführung
    rHinv = rHhat/rHtilde;
    rH = rHtilde*rHhatinv;

end

== matlab function libbha_kinetic_cc/lib_kin_inhom_S1 ==
  data: H_1h_w input size=[4,4]; dHdq_1h_w input size=[12,4]; r_Bik_1h input size=[4,3]; delta_F_ik_Pressure input size=[3,1]; tau output size=[3,1]
function tau   = ksim_kin_tau(H_1h_w, dHdq_1h_w, r_Bik_1h, delta_F_ik_Pressure)
% kinvsim_fav_4b2
    
    % Änderungen zut alten Version:
    % - Rückrechnung mit Offsets der 4. Dimension der Homogenen Transformation (HOxx)
    % - richtige Saturierung des Ausgangsdrucks (optional)
    % - Tensordarstellung vermieden (Vektoren oder Matrizen sofern möglich), daher auch mehr getrennte Variablen
    % - Zusammenfassung bei Berechnungen unter Ausnutzung von 0-Einträgen (schwerer lesbar und weniger allgemein, dafür schneller zu rechnen)

%% Kraftdifferenz (aktiv)

    F_active_d = delta_F_ik_Pressure;
    
%% Kinetische Vorwärtsrechnung

	% SI = ceil(max(linspace(1,9,9)'*ones(1,9),ones(9,1)*linspace(1,9,9))/3);
    t1a = zeros(3,1); 
    
    for row = 1:3
		rm = row - 1;
        
        for bi=1:3  
            t1a(row) = t1a(row) + (H_1h_w(:,3)*F_active_d(bi))' * dHdq_1h_w((1:4)+4*rm,:)*r_Bik_1h(:,bi);
        end
    end
    tau   = t1a;

end

== matlab function libbha_kinetic_cc/lib_kin_hom ==
  data: H_1h_w input size=[4,4]; H_2h_w input size=[4,4]; H_3h_w input size=[4,4]; dHdq_1h_w input size=[36,4]; dHdq_2h_w input size=[36,4]; dHdq_3h_w input size=[36,4]; r_Bik_1h input size=[4,3]; r_Bik_2h input size=[4,3]; r_Bik_3h input size=[4,3]; g_w input size=[3,1]; F_ik_Spring input size=[9,1]; F_ik_Damper input size=[9,1]; F_ik_Bending input size=[9,1]; PAR_M_i input size=[3,1]; B output size=[9,9]; Ns output size=[9,1]; Ng output size=[9,1]; Nb output size=[9,1]; Nd output size=[9,1]
function [B, Ns, Ng, Nb, Nd]  = ksim_kin_BN(H_1h_w, H_2h_w, H_3h_w, dHdq_1h_w, dHdq_2h_w, dHdq_3h_w, r_Bik_1h, r_Bik_2h, r_Bik_3h, g_w, F_ik_Spring, F_ik_Damper, F_ik_Bending, PAR_M_i)
% kinvsim_fav_4b2
    
    % Änderungen zut alten Version:
    % - Rückrechnung mit Offsets der 4. Dimension der Homogenen Transformation (HOxx)
    % - richtige Saturierung des Ausgangsdrucks (optional)
    % - Tensordarstellung vermieden (Vektoren oder Matrizen sofern möglich), daher auch mehr getrennte Variablen
    % - Zusammenfassung bei Berechnungen unter Ausnutzung von 0-Einträgen (schwerer lesbar und weniger allgemein, dafür schneller zu rechnen)

    g_w4 = [g_w; 0];

%% Kraftdifferenz (passiv)

   %F_passive   = F_ik_Spring + F_ik_Damper;
   %F_passive_d = F_passive - [F_passive(4:9); zeros(3,1)];
    F_Spring_d  = F_ik_Spring  - [F_ik_Spring(4:9);  zeros(3,1)];
    F_Damper_d  = F_ik_Damper  - [F_ik_Damper(4:9);  zeros(3,1)];
    F_Bending_d = F_ik_Bending - [F_ik_Bending(4:9); zeros(3,1)];
    
%% Kinetische Vorwärtsrechnung

	% SI = ceil(max(linspace(1,9,9)'*ones(1,9),ones(9,1)*linspace(1,9,9))/3);
    SI = [1 1 1 2 2 2 3 3 3;1 1 1 2 2 2 3 3 3;1 1 1 2 2 2 3 3 3;2 2 2 2 2 2 3 3 3;2 2 2 2 2 2 3 3 3;2 2 2 2 2 2 3 3 3;3 3 3 3 3 3 3 3 3;3 3 3 3 3 3 3 3 3;3 3 3 3 3 3 3 3 3];
    B1  = zeros(9,9); B2  = zeros(9,9); B3  = zeros(9,9);
    N1g = zeros(9,1); N2g = zeros(9,1); N3g = zeros(9,1);
   %N1p = zeros(9,1); N2p = zeros(9,1); N3p = zeros(9,1);
    N1s = zeros(9,1); N2s = zeros(9,1); N3s = zeros(9,1);
    N1b = zeros(9,1); N2b = zeros(9,1); N3b = zeros(9,1);
    N1d = zeros(9,1); N2d = zeros(9,1); N3d = zeros(9,1);
    
    for row = 1:9
		rm = row - 1;
        for col = 1:9
			cm = col - 1;
            B3(row,col) = dHdq_3h_w((1:4)+4*cm,4)'*dHdq_3h_w((1:4)+4*rm,4); % *PAR_M_i(3) am Ende
            if SI(row,col) <= 2
                B2(row,col) = dHdq_2h_w((1:4)+4*cm,4)'*dHdq_2h_w((1:4)+4*rm,4); % *PAR_M_i(2) am Ende
                if SI(row,col) <= 1
                    B1(row,col) = dHdq_1h_w((1:4)+4*cm,4)'*dHdq_1h_w((1:4)+4*rm,4); % *PAR_M_i(1) am Ende
                end
            end
        end
        N3g(row) = - g_w4'*dHdq_3h_w((1:4)+4*rm,4); % *PAR_M_i(3) am Ende
        if SI(row,1) <= 2
            N2g(row) = - g_w4'*dHdq_2h_w((1:4)+4*rm,4); % *PAR_M_i(2) am Ende
            if SI(row,1) <= 1
                N1g(row) = - g_w4'*dHdq_1h_w((1:4)+4*rm,4); % *PAR_M_i(1) am Ende
            end
        end
        
        for bi=1:3  
           %N3p(row) = N3p(row) + (H_3h_w(:,3)*F_passive_d(bi+6))' * dHdq_3h_w((1:4)+4*rm,:)*r_Bik_3h(:,bi);
            N3s(row) = N3s(row) + (H_3h_w(:,3)*F_Spring_d(bi+6))'  * dHdq_3h_w((1:4)+4*rm,:)*r_Bik_3h(:,bi);
            N3d(row) = N3d(row) + (H_3h_w(:,3)*F_Damper_d(bi+6))'  * dHdq_3h_w((1:4)+4*rm,:)*r_Bik_3h(:,bi);
            N3b(row) = N3b(row) + (H_3h_w(:,3)*F_Bending_d(bi+6))' * dHdq_3h_w((1:4)+4*rm,:)*r_Bik_3h(:,bi);
            if SI(row,1) <= 2
               %N2p(row) = N2p(row) + (H_2h_w(:,3)*F_passive_d(bi+3))' * dHdq_2h_w((1:4)+4*rm,:)*r_Bik_2h(:,bi);
                N2s(row) = N2s(row) + (H_2h_w(:,3)*F_Spring_d(bi+3))'  * dHdq_2h_w((1:4)+4*rm,:)*r_Bik_2h(:,bi);
                N2d(row) = N2d(row) + (H_2h_w(:,3)*F_Damper_d(bi+3))'  * dHdq_2h_w((1:4)+4*rm,:)*r_Bik_2h(:,bi);
                N2b(row) = N2b(row) + (H_2h_w(:,3)*F_Bending_d(bi+3))' * dHdq_2h_w((1:4)+4*rm,:)*r_Bik_2h(:,bi);
                if SI(row,1) <= 1
                   %N1p(row) = N1p(row) + (H_1h_w(:,3)*F_passive_d(bi))' * dHdq_1h_w((1:4)+4*rm,:)*r_Bik_1h(:,bi);
                    N1s(row) = N1s(row) + (H_1h_w(:,3)*F_Spring_d(bi))'  * dHdq_1h_w((1:4)+4*rm,:)*r_Bik_1h(:,bi);
                    N1d(row) = N1d(row) + (H_1h_w(:,3)*F_Damper_d(bi))'  * dHdq_1h_w((1:4)+4*rm,:)*r_Bik_1h(:,bi);
                    N1b(row) = N1b(row) + (H_1h_w(:,3)*F_Bending_d(bi))' * dHdq_1h_w((1:4)+4*rm,:)*r_Bik_1h(:,bi);
                end
            end 
        end
    end
    
    B    = B1*PAR_M_i(1)  + B2*PAR_M_i(2)  + B3*PAR_M_i(3);
    Ng   = N1g*PAR_M_i(1) + N2g*PAR_M_i(2) + N3g*PAR_M_i(3);
   %Np   = N1p + N2p + N3p;
    Ns   = N1s + N2s + N3s;
    Nd   = N1d + N2d + N3d;
    Nb   = N1b + N2b + N3b;

end

== matlab function libbha_kinetic_cc/lib_kin_inhom ==
  data: H_1h_w input size=[4,4]; H_2h_w input size=[4,4]; H_3h_w input size=[4,4]; dHdq_1h_w input size=[36,4]; dHdq_2h_w input size=[36,4]; dHdq_3h_w input size=[36,4]; r_Bik_1h input size=[4,3]; r_Bik_2h input size=[4,3]; r_Bik_3h input size=[4,3]; F_ik_Pressure input size=[9,1]; tau output size=[9,1]
function tau   = ksim_kin_tau(H_1h_w, H_2h_w, H_3h_w, dHdq_1h_w, dHdq_2h_w, dHdq_3h_w, r_Bik_1h, r_Bik_2h, r_Bik_3h, F_ik_Pressure)
% kinvsim_fav_4b2
    
    % Änderungen zut alten Version:
    % - Rückrechnung mit Offsets der 4. Dimension der Homogenen Transformation (HOxx)
    % - richtige Saturierung des Ausgangsdrucks (optional)
    % - Tensordarstellung vermieden (Vektoren oder Matrizen sofern möglich), daher auch mehr getrennte Variablen
    % - Zusammenfassung bei Berechnungen unter Ausnutzung von 0-Einträgen (schwerer lesbar und weniger allgemein, dafür schneller zu rechnen)

%% Kraftdifferenz (aktiv)

    F_active_d = F_ik_Pressure - [F_ik_Pressure(4:9); zeros(3,1)];
    
%% Kinetische Vorwärtsrechnung

	% SI = ceil(max(linspace(1,9,9)'*ones(1,9),ones(9,1)*linspace(1,9,9))/3);
    SI = [1 1 1 2 2 2 3 3 3;1 1 1 2 2 2 3 3 3;1 1 1 2 2 2 3 3 3;2 2 2 2 2 2 3 3 3;2 2 2 2 2 2 3 3 3;2 2 2 2 2 2 3 3 3;3 3 3 3 3 3 3 3 3;3 3 3 3 3 3 3 3 3;3 3 3 3 3 3 3 3 3];
    t1a = zeros(9,1); t2a = zeros(9,1); t3a = zeros(9,1);
    
    for row = 1:9
		rm = row - 1;
        
        for bi=1:3  
            t3a(row) = t3a(row) + (H_3h_w(:,3)*F_active_d(bi+6))' * dHdq_3h_w((1:4)+4*rm,:)*r_Bik_3h(:,bi);
            if SI(row,1) <= 2
                t2a(row) = t2a(row) + (H_2h_w(:,3)*F_active_d(bi+3))' * dHdq_2h_w((1:4)+4*rm,:)*r_Bik_2h(:,bi);
                if SI(row,1) <= 1
                    t1a(row) = t1a(row) + (H_1h_w(:,3)*F_active_d(bi))' * dHdq_1h_w((1:4)+4*rm,:)*r_Bik_1h(:,bi);
                end
            end 
        end
    end
    
    tau   = t1a + t2a + t3a;   

end
